simulink model "mconversionMuxInBus"  (Simulink 6.0)
settings: Solver=FixedStepDiscrete  StartTime=0.0  StopTime=10.0  RelTol=1e-3
undefined symbols (not defined in the file or in its folder): DiscIntNeverNeededParam
libraries: simulink x1
settings Model: Creator=awarlock  LastModifiedBy=awarlock  ExtModeAutoUpdateStatusClock=off

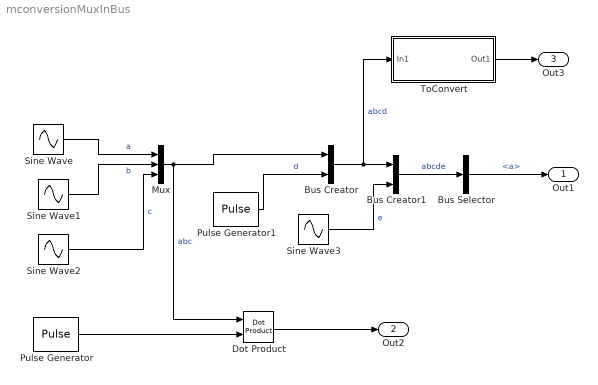
== system mconversionMuxInBus ==
  Bus Creator : BusCreator  DialogController=Simulink.DDGSource_Bus  Inputs=2
  Bus Creator1 : BusCreator  DialogController=Simulink.DDGSource_Bus  Inputs=2
  Bus Selector : BusSelector  DialogController=Simulink.DDGSource_Bus  OutputSignals=abcd.abc.a
  Dot Product : simulink/Math Operations/Dot Product  InputSameDT=on  OutDataType=sfix(16)  OutScaling=2^-10  DoSatur=off
  Mux : Mux  Inputs=3
  Pulse Generator : DiscretePulseGenerator  Amplitude=1:3  SampleTime=0.1
  Pulse Generator1 : DiscretePulseGenerator  Amplitude=1:3  SampleTime=0.1
  Sine Wave{,1..3} (4 alike) : Sin  SampleTime=0.1
  ToConvert : Subsystem  TreatAsAtomicUnit=on
  Out1 : Outport
  Out2 : Outport  Port=2
  Out3 : Outport  Port=3
  wires:
  Sine Wave/1 -> Mux/1  "a"
  Sine Wave1/1 -> Mux/2  "b"
  Sine Wave2/1 -> Mux/3  "c"
  Pulse Generator/1 -> Dot Product/2
  Mux/1 -> Bus Creator/1, Dot Product/1  "abc"
  Pulse Generator1/1 -> Bus Creator/2  "d"
  Sine Wave3/1 -> Bus Creator1/2  "e"
  Bus Creator/1 -> Bus Creator1/1, ToConvert/1(In1)  "abcd"
  Bus Creator1/1 -> Bus Selector/1  "abcde"
  Bus Selector/1 -> Out1/1  "<a>"
  Dot Product/1 -> Out2/1
  ToConvert/1(Out1) -> Out3/1

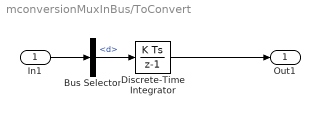
== system mconversionMuxInBus/ToConvert ==
  In1 : Inport  Port=1  LatchInput=off
  Bus Selector : BusSelector  DialogController=Simulink.DDGSource_Bus  OutputSignals=d
  Discrete-Time Integrator : DiscreteIntegrator  SampleTime=0.1  ICPrevOutput=DiscIntNeverNeededParam  ICPrevScaledInput=DiscIntNeverNeededParam
  Out1 : Outport
  wires:
  In1/1 -> Bus Selector/1
  Bus Selector/1 -> Discrete-Time Integrator/1  "<d>"
  Discrete-Time Integrator/1 -> Out1/1
